simulink model "PowertrainCoolingModel"  (R2020b)
settings: Solver=VariableStepAuto  StartTime=0.0  StopTime=Request.Scaled.Time(end)  MaxStep=1e-1  MinStep=1e-9  RelTol=1e-3
values from neighbouring files (symbols this model uses):
  Accumulator = StraightFinCalculations( Accumulator )    [PowertrainCoolingWrapper.m]
  Controller = StraightFinCalculations( Controller )    [PowertrainCoolingWrapper.m]
  Environment = EnvironmentCalculations( Environment )    [PowertrainCoolingWrapper.m]
  Motor = MotorCalculations( Motor )    [PowertrainCoolingWrapper.m]
  Request = RequestCalculations( Request, Data )    [PowertrainCoolingWrapper.m]
undefined symbols (not defined in the file or in its folder): Chassis, Material
libraries: fl_lib x54, nesl_utility x21
settings Model: Creator=bechr  LastModifiedBy=maxbo
settings SolverCC: InitialStep=1e-9  MaxConsecutiveMinStep=10
settings ModelReferenceCC: ModelReferenceMinAlgLoopOccurrences=on

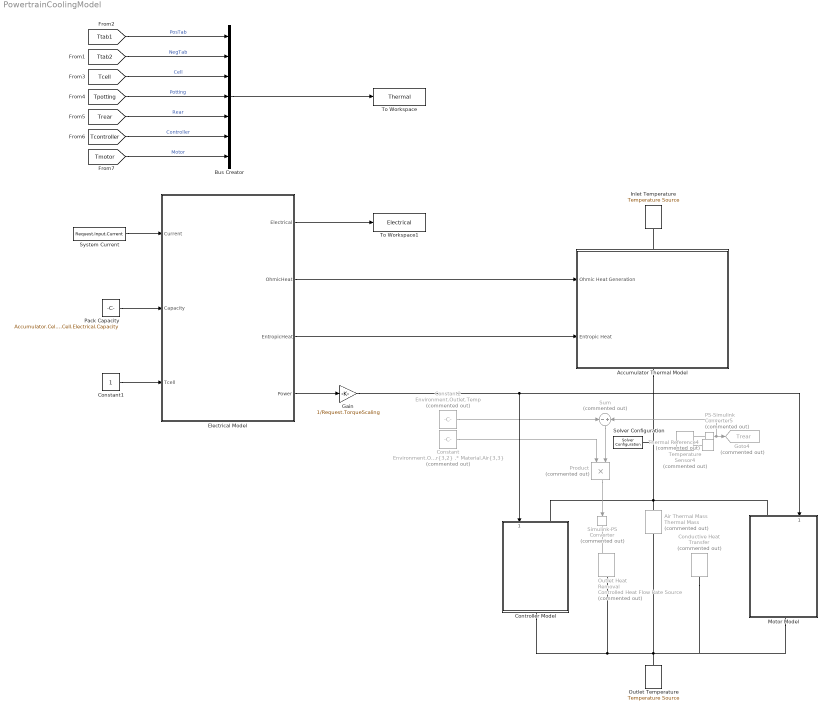
== system PowertrainCoolingModel ==
  Accumulator Thermal Model : Subsystem
      settings: PortSchema="{\"entries\":[{\"content\":{\"sides\":[{\"content\":{\"connectorIds\":[\"LConn1\"]},\"type\":\"ConnectorPlacement.EquallySpacedRectSide\",\"uuid\":\"047de4e7-8380-4083-a16a-e3dcc0474bf0\"},{\"content\":{\"connectorIds\":[\"RConn1\"],\"side\":\"RIGHT\"},\"type\":\"ConnectorPlacement.EquallySpacedRectSide\",\"uuid\":\"fb2ea971-3892-49c2-b754-190bbc105b65\"},{\"content\":{\"connectorIds\":[\"In1\",\"In2\"],\"side\":\"TOP\"},\"type\":\"ConnectorPlacement.EquallySpacedRectSide\",\"uuid\":\"52ae1223-76c9-471f-ad3e-c3ae8e976854\"}]},\"type\":\"ConnectorPlacement.EquallySpacedConnector\",\"uuid\":\"9beae297-ed97-4137-a2f6-556fb11424ca\"}],\"packageUris\":[\"http://schema.mathworks.com/mf0/Connector/19700101\"],\"version\":\"1.0\"}"
  Air Thermal Mass : fl_lib/Thermal/Thermal Elements/Thermal Mass  Commented=on  mass=0.995 .* Chassis.Dimensions.Volume kg  sp_heat=1.0090 kJ/kg/K  T_specify=on  T_priority=High  T=Environment.Outlet.Temp degC  T_nominal_specify=off  T_nominal_unit=K  T_nominal_value=1  Q_specify=off  Q_priority=None  Q=0 W  Q_nominal_specify=off  Q_nominal_unit=W  Q_nominal_value=1
  Bus Creator : BusCreator  Inputs=7
  Conductive Heat Transfer : fl_lib/Thermal/Thermal Elements/Conductive Heat Transfer  Commented=on  area=Chassis.Dimensions.Area m^2  thickness=Chassis.Dimensions.Thickness m  th_cond=Chassis.Thermal.k W/(m*K)  T_specify=off  T_priority=None  T=0 K  T_nominal_specify=off  T_nominal_unit=K  T_nominal_value=1  Q_specify=off  Q_priority=None  Q=0 W  Q_nominal_specify=off  Q_nominal_unit=W  Q_nominal_value=1
  Constant : Constant  Commented=on  Value=Environment.Outlet.FlowRate .* Material.Air{3,2} .* Material.Air{3,3}
  Constant1 : Constant
  Constant2 : Constant  Commented=on  Value=Environment.Outlet.Temp
  Controller Model : Subsystem
      settings: PortSchema="{\"entries\":[{\"content\":{\"sides\":[{\"content\":{\"connectorIds\":[\"LConn1\"]},\"type\":\"ConnectorPlacement.EquallySpacedRectSide\",\"uuid\":\"ee03d1dc-ccff-454a-ba9d-20e22337bc28\"},{\"content\":{\"connectorIds\":[\"In1\",\"RConn1\"],\"side\":\"RIGHT\"},\"type\":\"ConnectorPlacement.EquallySpacedRectSide\",\"uuid\":\"b1e6da54-ab19-4ef3-af09-0565bd1c2c81\"},{\"content\":{\"connectorIds\":[],\"side\":\"TOP\"},\"type\":\"ConnectorPlacement.EquallySpacedRectSide\",\"uuid\":\"cc30cdce-b0f9-4be0-bd93-6142d7ef4c72\"}]},\"type\":\"ConnectorPlacement.EquallySpacedConnector\",\"uuid\":\"1c37dcd3-68ba-409f-82c7-20e952dc67e1\"}],\"packageUris\":[\"http://schema.mathworks.com/mf0/Connector/19700101\"],\"version\":\"1.0\"}"
  Electrical Model : Subsystem
  Gain : Gain  Gain=1/Request.TorqueScaling
  Goto4 : Goto  Commented=on  GotoTag=Trear  TagVisibility=global
  Inlet Temperature : fl_lib/Thermal/Thermal Sources/Temperature Source  temperature=Environment.Inlet.Temp degC
  Motor Model : Subsystem
      settings: PortSchema="{\"entries\":[{\"content\":{\"sides\":[{\"content\":{\"connectorIds\":[\"LConn1\"]},\"type\":\"ConnectorPlacement.EquallySpacedRectSide\",\"uuid\":\"ee03d1dc-ccff-454a-ba9d-20e22337bc28\"},{\"content\":{\"connectorIds\":[\"RConn1\",\"In1\"],\"side\":\"RIGHT\"},\"type\":\"ConnectorPlacement.EquallySpacedRectSide\",\"uuid\":\"b1e6da54-ab19-4ef3-af09-0565bd1c2c81\"},{\"content\":{\"connectorIds\":[],\"side\":\"TOP\"},\"type\":\"ConnectorPlacement.EquallySpacedRectSide\",\"uuid\":\"cc30cdce-b0f9-4be0-bd93-6142d7ef4c72\"}]},\"type\":\"ConnectorPlacement.EquallySpacedConnector\",\"uuid\":\"1c37dcd3-68ba-409f-82c7-20e952dc67e1\"}],\"packageUris\":[\"http://schema.mathworks.com/mf0/Connector/19700101\"],\"version\":\"1.0\"}"
  Outlet Temperature : fl_lib/Thermal/Thermal Sources/Temperature Source  temperature=Environment.Outlet.Temp degC
  Outlet Heat Removal : fl_lib/Thermal/Thermal Sources/Controlled Heat Flow Rate Source  Commented=on
  PS-Simulink Converter5 : nesl_utility/PS-Simulink Converter  Commented=on  PhysicalDomain=network_engine_domain  SubClassName=ps_output  LeftPortType=input  RightPortType=output  PseudoPeriodic=off  Frequencies=[]  Unit=inherit  AffineConversion=off
  Pack Capacity : Constant  Value=Accumulator.Cell.Electrical.NCells .* Accumulator.Cell.Electrical.Capacity
  Product : Product  Commented=on
  Simulink-PS Converter : nesl_utility/Simulink-PS Converter  Commented=on  PhysicalDomain=network_engine_domain  SubClassName=ps_input  LeftPortType=input  RightPortType=output  PseudoPeriodic=off  Frequencies=[]  NoiseDistribution=none  NoiseParameters=[]  Unit=1  AffineConversion=off  FilteringAndDerivatives=provide  SimscapeFilterOrder=1  InputFilterTimeConstant=0.001  UdotUserProvided=0
  Solver Configuration : nesl_utility/Solver Configuration  PhysicalDomain=network_engine_domain  SubClassName=solver  LeftPortType=input  RightPortType=generic  Tones=[]  Harmonics=[]  SimulateNoise=off  Profile=off  UseLocalSampling=off  EnableSwitchedLinearOptims=on  FrequencyDomain=off  UseCCode=off  RelTol=0.001  AbsTol=1e-06  MinStep=1e-09  ToWorkspace=off  RevertToSquareIcSolve=off  NumHomotopyIterations=100  PhasorMode=off  PhasorModeNumHarmonics=1  DoDC=on  ResidualTolerance=1e-09  UseLocalSolver=off  LocalSolverChoice=NE_BACKWARD_EULER_ADVANCER  LocalSolverSampleTime=0.001  DoFixedCost=off  MaxNonlinIter=3  MaxModeIter=2  ComputeImpulses=off  ImpulseIterations=2  LinearAlgebra=auto  EquationFormulation=NE_TIME_EF  DelaysMemoryBudget=1024  AutomaticFiltering=on  FilteringTimeConstant=0.001  PartitionStorageMethod=AS_NEEDED  PartitionMemoryBudget=1024  PartitionMethod=ROBUST
  Sum : Sum  Commented=on  Inputs=-|+
  System Current : FromWorkspace  VariableName=Request.Input.Current  OutputAfterFinalValue=Setting to zero
  Temperature Sensor4 : fl_lib/Thermal/Thermal Sensors/Temperature Sensor  Commented=on
  Thermal Reference4 : fl_lib/Thermal/Thermal Elements/Thermal Reference  Commented=on
  To Workspace : ToWorkspace  VariableName=Thermal  SaveFormat=Timeseries  SampleTime=-1
  To Workspace1 : ToWorkspace  VariableName=Electrical  SaveFormat=Timeseries  SampleTime=-1
  wires:
  [Ttab1] -> Bus Creator/1  "PosTab"
  [Tcell] -> Bus Creator/3  "Cell"
  [Ttab2] -> Bus Creator/2  "NegTab"
  [Tpotting] -> Bus Creator/4  "Potting"
  [Trear] -> Bus Creator/5  "Rear"
  [Tcontroller] -> Bus Creator/6  "Controller"
  [Tmotor] -> Bus Creator/7  "Motor"
  Bus Creator/1 -> To Workspace/1
  Electrical Model/4(Power) -> Gain/1
  System Current/1 -> Electrical Model/1(Current)
  Pack Capacity/1 -> Electrical Model/2(Capacity)
  Electrical Model/1(Electrical) -> To Workspace1/1
  Electrical Model/2(OhmicHeat) -> Accumulator Thermal Model/1(Ohmic Heat Generation)
  Electrical Model/3(EntropicHeat) -> Accumulator Thermal Model/2(" Entropic Heat")
  Constant1/1 -> Electrical Model/3(Tcell)
  Constant2/1 -> Sum/1
  PS-Simulink Converter5/1 -> Sum/2, Goto4/1
  Product/1 -> Simulink-PS Converter/1
  Sum/1 -> Product/2
  Constant/1 -> Product/1
  Gain/1 -> Motor Model/1("Accumulator Power "), Controller Model/1("Accumulator Power ")
  connections:
  Simulink-PS Converter/RConn1 -- Outlet Heat Removal/RConn1
  Outlet Temperature/LConn1 -- Solver Configuration/RConn1 -- Accumulator Thermal Model/RConn1 -- Motor Model/RConn1 -- Controller Model/RConn1 -- Controller Model/LConn1 -- Outlet Heat Removal/LConn1 -- Conductive Heat Transfer/RConn1 -- Motor Model/LConn1
  Thermal Reference4/LConn1 -- Temperature Sensor4/RConn1
  PS-Simulink Converter5/LConn1 -- Temperature Sensor4/RConn2
  Accumulator Thermal Model/LConn1 -- Inlet Temperature/LConn1

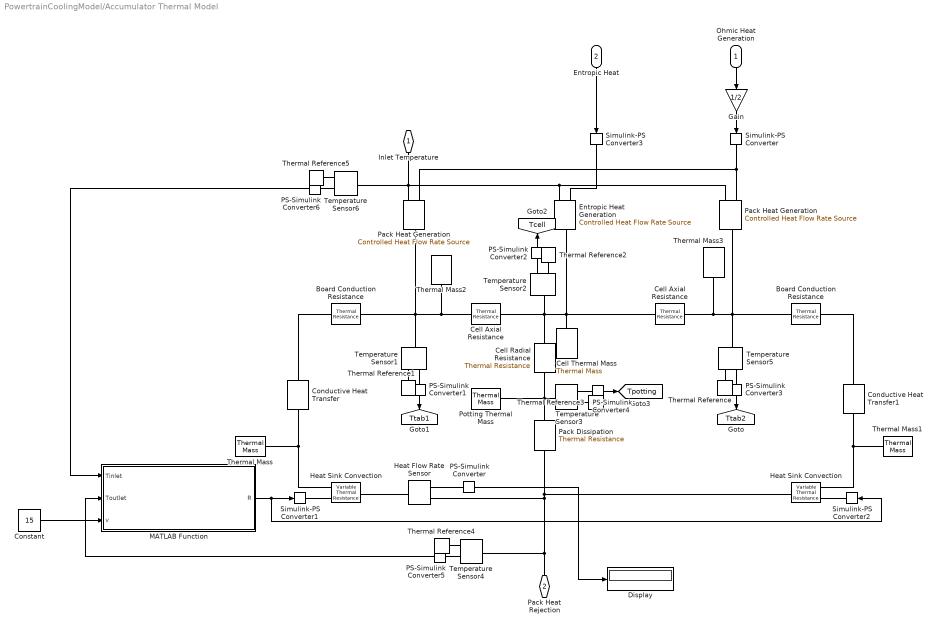
== system PowertrainCoolingModel/Accumulator Thermal Model ==
  Ohmic Heat Generation : Inport
  " Entropic Heat" : Inport  Port=2
  "    Pack Heat Generation" : fl_lib/Thermal/Thermal Sources/Controlled Heat Flow Rate Source
  "  Pack Heat Generation" : fl_lib/Thermal/Thermal Sources/Controlled Heat Flow Rate Source
  Board Conduction Resistance : fl_lib/Thermal/Thermal Elements/Thermal Resistance  resistance=Accumulator.Collector.Thermal.Resistance K/W  T_specify=off  T_priority=None  T=0 K  T_nominal_specify=off  T_nominal_unit=K  T_nominal_value=1  Q_specify=off  Q_priority=None  Q=0 W  Q_nominal_specify=off  Q_nominal_unit=W  Q_nominal_value=1
      settings: SourceProductBaseCode=SS
  "Board Conduction Resistance " : fl_lib/Thermal/Thermal Elements/Thermal Resistance  resistance=1000000 K/W  T_specify=off  T_priority=None  T=0 K  T_nominal_specify=off  T_nominal_unit=K  T_nominal_value=1  Q_specify=off  Q_priority=None  Q=0 W  Q_nominal_specify=off  Q_nominal_unit=W  Q_nominal_value=1
      settings: SourceProductBaseCode=SS
  Cell Axial Resistance : fl_lib/Thermal/Thermal Elements/Thermal Resistance  resistance=Accumulator.Cell.Thermal.R_Axial K/W  T_specify=off  T_priority=None  T=0 K  T_nominal_specify=off  T_nominal_unit=K  T_nominal_value=1  Q_specify=off  Q_priority=None  Q=0 W  Q_nominal_specify=off  Q_nominal_unit=W  Q_nominal_value=1
      settings: SourceProductBaseCode=SS
  "Cell Axial Resistance " : fl_lib/Thermal/Thermal Elements/Thermal Resistance  resistance=Accumulator.Cell.Thermal.R_Axial K/W  T_specify=off  T_priority=None  T=0 K  T_nominal_specify=off  T_nominal_unit=K  T_nominal_value=1  Q_specify=off  Q_priority=None  Q=0 W  Q_nominal_specify=off  Q_nominal_unit=W  Q_nominal_value=1
      settings: SourceProductBaseCode=SS
  Cell Radial Resistance : fl_lib/Thermal/Thermal Elements/Thermal Resistance  resistance=Accumulator.Cell.Thermal.R_Radial K/W  T_specify=off  T_priority=None  T=0 K  T_nominal_specify=off  T_nominal_unit=K  T_nominal_value=1  Q_specify=off  Q_priority=None  Q=0 W  Q_nominal_specify=off  Q_nominal_unit=W  Q_nominal_value=1
      settings: SourceProductBaseCode=SS
  Cell Thermal Mass : fl_lib/Thermal/Thermal Elements/Thermal Mass  mass=Accumulator.Cell.Electrical.NCells .* Accumulator.Cell.Mass.m kg  sp_heat=Accumulator.Cell.Thermal.cp kJ/kg/K  T_specify=on  T_priority=Low  T=Environment.Inlet.Temp degC  T_nominal_specify=off  T_nominal_unit=K  T_nominal_value=1  Q_specify=off  Q_priority=None  Q=0 W  Q_nominal_specify=off  Q_nominal_unit=W  Q_nominal_value=1
  Conductive Heat Transfer : fl_lib/Thermal/Thermal Elements/Conductive Heat Transfer  area=Accumulator.Fin.Dimensions.Width * Accumulator.Fin.Dimensions.Length * 5 m^2  thickness=0.2 mm  th_cond=1.6 W/(m*K)  T_specify=off  T_priority=None  T=0 K  T_nominal_specify=off  T_nominal_unit=K  T_nominal_value=1  Q_specify=off  Q_priority=None  Q=0 W  Q_nominal_specify=off  Q_nominal_unit=W  Q_nominal_value=1
  Conductive Heat Transfer1 : fl_lib/Thermal/Thermal Elements/Conductive Heat Transfer  area=Accumulator.Fin.Dimensions.Width * Accumulator.Fin.Dimensions.Length * 5 m^2  thickness=0.2 mm  th_cond=1.6 W/(m*K)  T_specify=off  T_priority=None  T=0 K  T_nominal_specify=off  T_nominal_unit=K  T_nominal_value=1  Q_specify=off  Q_priority=None  Q=0 W  Q_nominal_specify=off  Q_nominal_unit=W  Q_nominal_value=1
  Constant : Constant  Value=15
  Display : Display
  Entropic Heat Generation : fl_lib/Thermal/Thermal Sources/Controlled Heat Flow Rate Source
  Gain : Gain  Gain=1/2
  Heat Flow Rate Sensor : fl_lib/Thermal/Thermal Sensors/Heat Flow Rate Sensor
      settings: SourceProductBaseCode=SS
  Heat Sink Convection : fl_lib/Thermal/Thermal Elements/Variable Thermal Resistance  R_min=0 K/W  T_specify=off  T_priority=None  T=0 K  T_nominal_specify=off  T_nominal_unit=K  T_nominal_value=1  Q_specify=off  Q_priority=None  Q=0 W  Q_nominal_specify=off  Q_nominal_unit=W  Q_nominal_value=1
      settings: SourceProductBaseCode=SS  InternalSimscapePortConfiguration="{\"Bottom\":[],\"Left\":[{\"id\":\"A\",\"label\":\"A\",\"type\":\"foundation.thermal.thermal\"},{\"id\":\"R\",\"label\":\"R\",\"type\":\"input\"}],\"Right\":[{\"id\":\"B\",\"label\":\"B\",\"type\":\"foundation.thermal.thermal\"}],\"Top\":[]}"
  "Heat Sink Convection " : fl_lib/Thermal/Thermal Elements/Variable Thermal Resistance  R_min=0 K/W  T_specify=off  T_priority=None  T=0 K  T_nominal_specify=off  T_nominal_unit=K  T_nominal_value=1  Q_specify=off  Q_priority=None  Q=0 W  Q_nominal_specify=off  Q_nominal_unit=W  Q_nominal_value=1
      settings: SourceProductBaseCode=SS  InternalSimscapePortConfiguration="{\"Bottom\":[],\"Left\":[{\"id\":\"A\",\"label\":\"A\",\"type\":\"foundation.thermal.thermal\"},{\"id\":\"R\",\"label\":\"R\",\"type\":\"input\"}],\"Right\":[{\"id\":\"B\",\"label\":\"B\",\"type\":\"foundation.thermal.thermal\"}],\"Top\":[]}"
  MATLAB Function : MATLAB Function  TreatAsAtomicUnit=on
  PS-Simulink Converter{,1..6} (7 alike) : nesl_utility/PS-Simulink Converter  PhysicalDomain=network_engine_domain  SubClassName=ps_output  LeftPortType=input  RightPortType=output  PseudoPeriodic=off  Frequencies=[]  Unit=inherit  AffineConversion=off
  Pack Dissipation : fl_lib/Thermal/Thermal Elements/Thermal Resistance  resistance=1E6 K/W  T_specify=off  T_priority=None  T=0 K  T_nominal_specify=off  T_nominal_unit=K  T_nominal_value=1  Q_specify=off  Q_priority=None  Q=0 W  Q_nominal_specify=off  Q_nominal_unit=W  Q_nominal_value=1
      settings: SourceProductBaseCode=SS
  Potting Thermal Mass : fl_lib/Thermal/Thermal Elements/Thermal Mass  mass=Accumulator.Potting.Mass.m kg  sp_heat=Accumulator.Potting.Thermal.cp kJ/kg/K  T_specify=on  T_priority=Low  T=Environment.Inlet.Temp degC  T_nominal_specify=off  T_nominal_unit=K  T_nominal_value=1  Q_specify=off  Q_priority=None  Q=0 W  Q_nominal_specify=off  Q_nominal_unit=W  Q_nominal_value=1
  Simulink-PS Converter{,1..3} (4 alike) : nesl_utility/Simulink-PS Converter  PhysicalDomain=network_engine_domain  SubClassName=ps_input  LeftPortType=input  RightPortType=output  PseudoPeriodic=off  Frequencies=[]  NoiseDistribution=none  NoiseParameters=[]  Unit=1  AffineConversion=off  FilteringAndDerivatives=provide  SimscapeFilterOrder=1  InputFilterTimeConstant=0.001  UdotUserProvided=0
  Temperature Sensor{1..6} (6 alike) : fl_lib/Thermal/Thermal Sensors/Temperature Sensor
  Thermal Mass : fl_lib/Thermal/Thermal Elements/Thermal Mass  mass=1.16 / 2 * 5 kg  sp_heat=900 J/kg/K  T_specify=off  T_priority=High  T=300 K  T_nominal_specify=off  T_nominal_unit=K  T_nominal_value=1  Q_specify=off  Q_priority=None  Q=0 W  Q_nominal_specify=off  Q_nominal_unit=W  Q_nominal_value=1
  Thermal Mass1 : fl_lib/Thermal/Thermal Elements/Thermal Mass  mass=1.16 / 2 * 5 kg  sp_heat=900 J/kg/K  T_specify=off  T_priority=High  T=300 K  T_nominal_specify=off  T_nominal_unit=K  T_nominal_value=1  Q_specify=off  Q_priority=None  Q=0 W  Q_nominal_specify=off  Q_nominal_unit=W  Q_nominal_value=1
  Thermal Mass2 : fl_lib/Thermal/Thermal Elements/Thermal Mass  mass=2 * Accumulator.Cell.Electrical.NCells g  sp_heat=475 J/kg/K  T_specify=off  T_priority=High  T=300 K  T_nominal_specify=off  T_nominal_unit=K  T_nominal_value=1  Q_specify=off  Q_priority=None  Q=0 W  Q_nominal_specify=off  Q_nominal_unit=W  Q_nominal_value=1
  Thermal Mass3 : fl_lib/Thermal/Thermal Elements/Thermal Mass  mass=2 * Accumulator.Cell.Electrical.NCells g  sp_heat=475 J/kg/K  T_specify=off  T_priority=High  T=300 K  T_nominal_specify=off  T_nominal_unit=K  T_nominal_value=1  Q_specify=off  Q_priority=None  Q=0 W  Q_nominal_specify=off  Q_nominal_unit=W  Q_nominal_value=1
  Thermal Reference{,1..5} (6 alike) : fl_lib/Thermal/Thermal Elements/Thermal Reference
  " Inlet Temperature" : PMIOPort  Side=Left
  Pack Heat Rejection : PMIOPort  Port=2  Side=Right
  tag scope: Tcell=global, Tpotting=global, Ttab1=global, Ttab2=global
  wires:
  PS-Simulink Converter4/1 -> [Tpotting]
  PS-Simulink Converter3/1 -> [Ttab2]
  PS-Simulink Converter2/1 -> [Tcell]
  PS-Simulink Converter1/1 -> [Ttab1]
  Ohmic Heat Generation/1 -> Gain/1
  Gain/1 -> Simulink-PS Converter/1
  MATLAB Function/1(R) -> Simulink-PS Converter2/1, Simulink-PS Converter1/1
  PS-Simulink Converter5/1 -> MATLAB Function/2(Toutlet)
  PS-Simulink Converter6/1 -> MATLAB Function/1(Tinlet)
  Constant/1 -> MATLAB Function/3(v)
  " Entropic Heat"/1 -> Simulink-PS Converter3/1
  PS-Simulink Converter/1 -> Display/1
  connections:
  Temperature Sensor2/LConn1 -- Entropic Heat Generation/LConn1 -- Cell Thermal Mass/LConn1 -- "Cell Axial Resistance "/RConn1 -- Cell Radial Resistance/LConn1 -- Cell Axial Resistance/RConn1
  Temperature Sensor3/LConn1 -- Cell Radial Resistance/RConn1 -- Pack Dissipation/LConn1 -- Potting Thermal Mass/LConn1
  Conductive Heat Transfer/LConn1 -- Board Conduction Resistance/RConn1
  Heat Sink Convection/LConn1 -- Conductive Heat Transfer/RConn1 -- Thermal Mass/LConn1
  Thermal Reference1/LConn1 -- Temperature Sensor1/RConn1
  Temperature Sensor1/LConn1 -- Cell Axial Resistance/LConn1 -- Thermal Mass2/LConn1 -- "    Pack Heat Generation"/LConn1 -- Board Conduction Resistance/LConn1
  "Heat Sink Convection "/LConn1 -- Conductive Heat Transfer1/RConn1 -- Thermal Mass1/LConn1
  "    Pack Heat Generation"/RConn2 -- " Inlet Temperature"/RConn1 -- "  Pack Heat Generation"/RConn2 -- Entropic Heat Generation/RConn2 -- Temperature Sensor6/LConn1
  PS-Simulink Converter2/LConn1 -- Temperature Sensor2/RConn2
  "  Pack Heat Generation"/LConn1 -- Thermal Mass3/LConn1 -- "Cell Axial Resistance "/LConn1 -- Temperature Sensor5/LConn1 -- "Board Conduction Resistance "/LConn1
  PS-Simulink Converter3/LConn1 -- Temperature Sensor5/RConn2
  Thermal Reference/LConn1 -- Temperature Sensor5/RConn1
  Pack Dissipation/RConn1 -- Heat Flow Rate Sensor/RConn2 -- Temperature Sensor4/LConn1 -- Pack Heat Rejection/RConn1 -- "Heat Sink Convection "/RConn1
  "    Pack Heat Generation"/RConn1 -- Simulink-PS Converter/RConn1 -- "  Pack Heat Generation"/RConn1
  Conductive Heat Transfer1/LConn1 -- "Board Conduction Resistance "/RConn1
  PS-Simulink Converter4/LConn1 -- Temperature Sensor3/RConn2
  Thermal Reference3/LConn1 -- Temperature Sensor3/RConn1
  PS-Simulink Converter1/LConn1 -- Temperature Sensor1/RConn2
  Thermal Reference2/LConn1 -- Temperature Sensor2/RConn1
  Simulink-PS Converter1/RConn1 -- Heat Sink Convection/LConn2
  Thermal Reference4/LConn1 -- Temperature Sensor4/RConn1
  PS-Simulink Converter5/LConn1 -- Temperature Sensor4/RConn2
  PS-Simulink Converter6/LConn1 -- Temperature Sensor6/RConn2
  Thermal Reference5/LConn1 -- Temperature Sensor6/RConn1
  Simulink-PS Converter2/RConn1 -- "Heat Sink Convection "/LConn2
  Simulink-PS Converter3/RConn1 -- Entropic Heat Generation/RConn1
  Heat Flow Rate Sensor/LConn1 -- Heat Sink Convection/RConn1
  PS-Simulink Converter/LConn1 -- Heat Flow Rate Sensor/RConn1

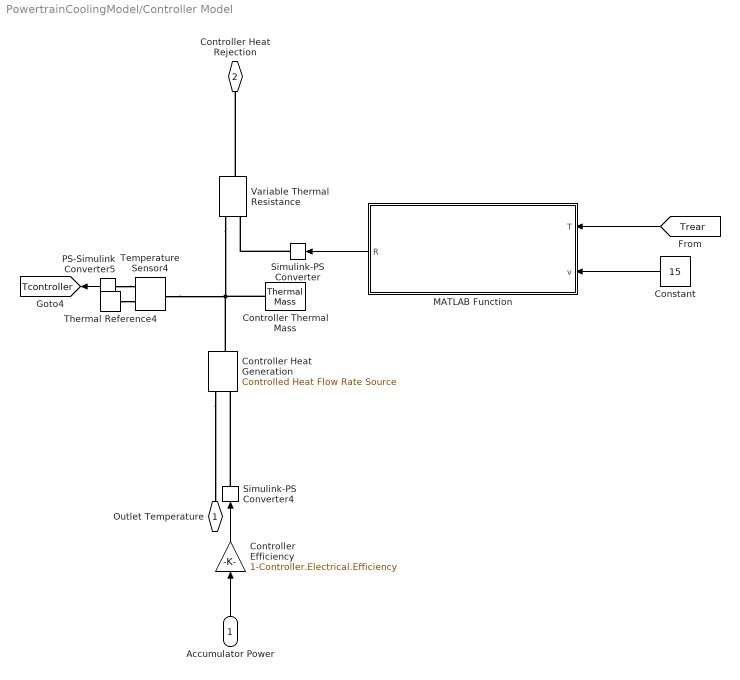
== system PowertrainCoolingModel/Controller Model ==
  "Accumulator Power " : Inport
  Constant : Constant  Value=15
  Controller Efficiency : Gain  Gain=1-Controller.Electrical.Efficiency
  Controller Heat Generation : fl_lib/Thermal/Thermal Sources/Controlled Heat Flow Rate Source
  Controller Thermal Mass : fl_lib/Thermal/Thermal Elements/Thermal Mass  mass=1 kg  sp_heat=2.2137e+03 J/kg/K  T_specify=on  T_priority=None  T=Environment.Outlet.Temp degC  T_nominal_specify=off  T_nominal_unit=K  T_nominal_value=1  Q_specify=off  Q_priority=None  Q=0 W  Q_nominal_specify=off  Q_nominal_unit=W  Q_nominal_value=1
  MATLAB Function : MATLAB Function  TreatAsAtomicUnit=on
  PS-Simulink Converter5 : nesl_utility/PS-Simulink Converter  PhysicalDomain=network_engine_domain  SubClassName=ps_output  LeftPortType=input  RightPortType=output  PseudoPeriodic=off  Frequencies=[]  Unit=inherit  AffineConversion=off
  Simulink-PS Converter : nesl_utility/Simulink-PS Converter  PhysicalDomain=network_engine_domain  SubClassName=ps_input  LeftPortType=input  RightPortType=output  PseudoPeriodic=off  Frequencies=[]  NoiseDistribution=none  NoiseParameters=[]  Unit=1  AffineConversion=off  FilteringAndDerivatives=provide  SimscapeFilterOrder=1  InputFilterTimeConstant=0.001  UdotUserProvided=0
  Simulink-PS Converter4 : nesl_utility/Simulink-PS Converter  PhysicalDomain=network_engine_domain  SubClassName=ps_input  LeftPortType=input  RightPortType=output  PseudoPeriodic=off  Frequencies=[]  NoiseDistribution=none  NoiseParameters=[]  Unit=1  AffineConversion=off  FilteringAndDerivatives=provide  SimscapeFilterOrder=1  InputFilterTimeConstant=0.001  UdotUserProvided=0
  Temperature Sensor4 : fl_lib/Thermal/Thermal Sensors/Temperature Sensor
  Thermal Reference4 : fl_lib/Thermal/Thermal Elements/Thermal Reference
  Variable Thermal Resistance : fl_lib/Thermal/Thermal Elements/Variable Thermal Resistance  R_min=0 K/W  T_specify=off  T_priority=None  T=0 K  T_nominal_specify=off  T_nominal_unit=K  T_nominal_value=1  Q_specify=off  Q_priority=None  Q=0 W  Q_nominal_specify=off  Q_nominal_unit=W  Q_nominal_value=1
      settings: SourceProductBaseCode=SS  InternalSimscapePortConfiguration="{\"Bottom\":[],\"Left\":[{\"id\":\"A\",\"label\":\"A\",\"type\":\"foundation.thermal.thermal\"},{\"id\":\"R\",\"label\":\"R\",\"type\":\"input\"}],\"Right\":[{\"id\":\"B\",\"label\":\"B\",\"type\":\"foundation.thermal.thermal\"}],\"Top\":[]}"
  Outlet Temperature : PMIOPort  Side=Left
  Controller Heat Rejection : PMIOPort  Port=2  Side=Right
  tag scope: Tcontroller=global
  wires:
  PS-Simulink Converter5/1 -> [Tcontroller]
  "Accumulator Power "/1 -> Controller Efficiency/1
  Controller Efficiency/1 -> Simulink-PS Converter4/1
  Constant/1 -> MATLAB Function/2(v)
  [Trear] -> MATLAB Function/1(T)
  MATLAB Function/1(R) -> Simulink-PS Converter/1
  connections:
  Controller Heat Generation/LConn1 -- Variable Thermal Resistance/LConn1 -- Temperature Sensor4/LConn1 -- Controller Thermal Mass/LConn1
  Simulink-PS Converter4/RConn1 -- Controller Heat Generation/RConn1
  Variable Thermal Resistance/RConn1 -- Controller Heat Rejection/RConn1
  Controller Heat Generation/RConn2 -- Outlet Temperature/RConn1
  PS-Simulink Converter5/LConn1 -- Temperature Sensor4/RConn2
  Thermal Reference4/LConn1 -- Temperature Sensor4/RConn1
  Simulink-PS Converter/RConn1 -- Variable Thermal Resistance/LConn2

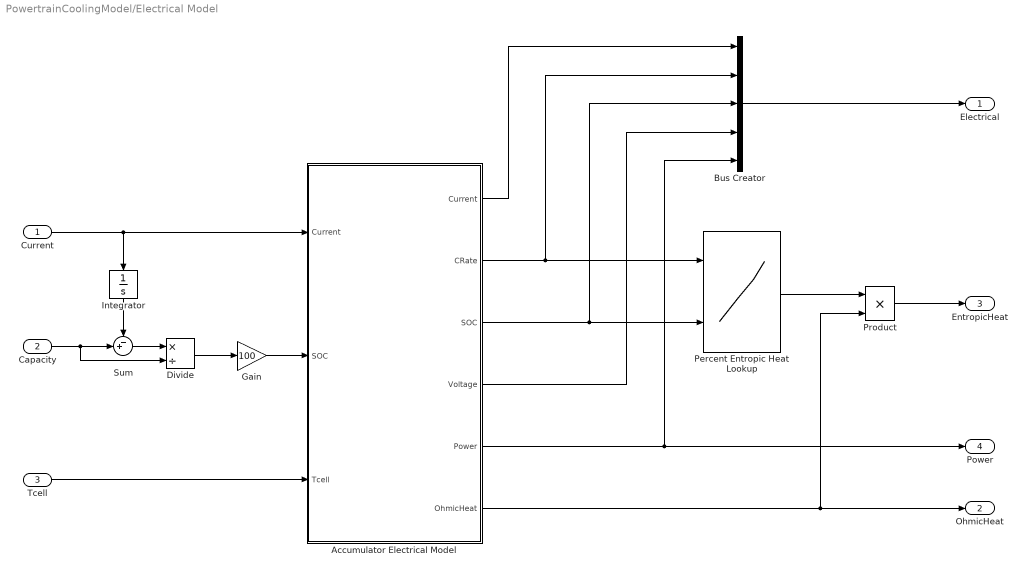
== system PowertrainCoolingModel/Electrical Model ==
  Current : Inport
  Capacity : Inport  Port=2
  Tcell : Inport  Port=3
  Accumulator Electrical Model : MATLAB Function  TreatAsAtomicUnit=on
  Bus Creator : BusCreator  Inputs=5
  Divide : Product  Inputs=*/
  Gain : Gain  Gain=100
  Integrator : Integrator
  Percent Entropic Heat Lookup : Lookup_n-D  BreakpointsForDimension1=Accumulator.Cell.Thermal.EntropyData.CRate  BreakpointsForDimension2=Accumulator.Cell.Thermal.EntropyData.SOC  BeginIndexSearchUsingPreviousIndexResult=on  Table=Accumulator.Cell.Thermal.EntropyData.PerEntropy  ExtrapMethod=Clip  DiagnosticForOutOfRangeInput=Warning  InternalRulePriority=Speed  RndMeth=Simplest  InputSameDT=on
      settings: InputPortMap=u0,u1
  Product : Product
  Sum : Sum  Inputs=-+|
  Electrical : Outport
  OhmicHeat : Outport  Port=2
  EntropicHeat : Outport  Port=3
  Power : Outport  Port=4
  wires:
  Accumulator Electrical Model/1(Current) -> Bus Creator/1
  Integrator/1 -> Sum/1
  Tcell/1 -> Accumulator Electrical Model/3(Tcell)
  Accumulator Electrical Model/6(OhmicHeat) -> Product/2, OhmicHeat/1
  Accumulator Electrical Model/2(CRate) -> Bus Creator/2, Percent Entropic Heat Lookup/1
  Capacity/1 -> Divide/2, Sum/2
  Accumulator Electrical Model/5(Power) -> Bus Creator/5, Power/1
  Current/1 -> Integrator/1, Accumulator Electrical Model/1("Current ")
  Accumulator Electrical Model/3(SOC) -> Bus Creator/3, Percent Entropic Heat Lookup/2
  Product/1 -> EntropicHeat/1
  Percent Entropic Heat Lookup/1 -> Product/1
  Accumulator Electrical Model/4(Voltage) -> Bus Creator/4
  Bus Creator/1 -> Electrical/1
  Sum/1 -> Divide/1
  Divide/1 -> Gain/1
  Gain/1 -> Accumulator Electrical Model/2("SOC ")

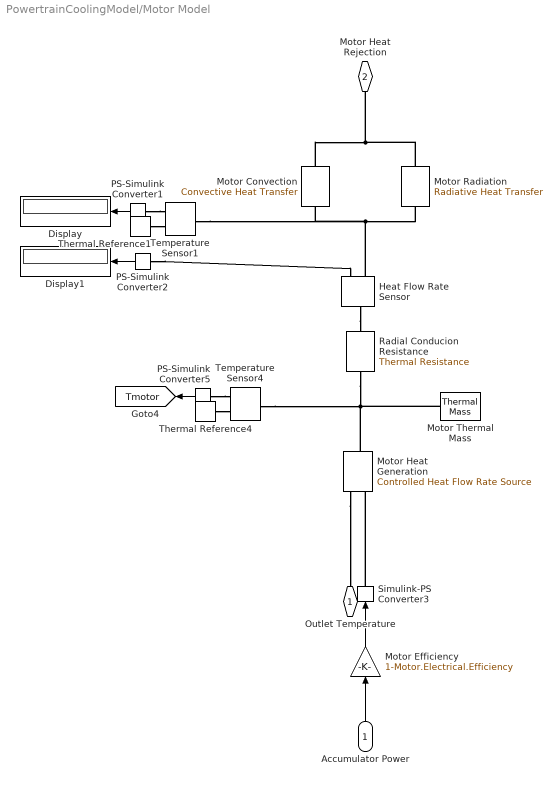
== system PowertrainCoolingModel/Motor Model ==
  "Accumulator Power " : Inport
  " Motor Heat Generation" : fl_lib/Thermal/Thermal Sources/Controlled Heat Flow Rate Source
  Display : Display
  Display1 : Display
  Heat Flow Rate Sensor : fl_lib/Thermal/Thermal Sensors/Heat Flow Rate Sensor
      settings: SourceProductBaseCode=SS
  Motor Convection : fl_lib/Thermal/Thermal Elements/Convective Heat Transfer  area=Motor.Dimensions.A m^2  heat_tr_coeff=Motor.Thermal.h W/(m^2 * K)  T_specify=off  T_priority=None  T=0 K  T_nominal_specify=off  T_nominal_unit=K  T_nominal_value=1  Q_specify=off  Q_priority=None  Q=0 W  Q_nominal_specify=off  Q_nominal_unit=W  Q_nominal_value=1
  Motor Efficiency : Gain  Gain=1-Motor.Electrical.Efficiency
  Motor Radiation : fl_lib/Thermal/Thermal Elements/Radiative Heat Transfer  area=Motor.Dimensions.A m^2  rad_tr_coeff=Motor.Thermal.eps W/(m^2*K^4)  T_specify=off  T_priority=None  T=0 K  T_nominal_specify=off  T_nominal_unit=K  T_nominal_value=1  Q_specify=off  Q_priority=None  Q=0 W  Q_nominal_specify=off  Q_nominal_unit=W  Q_nominal_value=1
      settings: SourceProductBaseCode=SS  InternalSimscapePortConfiguration="{\"Bottom\":[],\"Left\":[{\"id\":\"A\",\"label\":\"A\",\"type\":\"foundation.thermal.thermal\"}],\"Right\":[{\"id\":\"B\",\"label\":\"B\",\"type\":\"foundation.thermal.thermal\"}],\"Top\":[]}"
  Motor Thermal Mass : fl_lib/Thermal/Thermal Elements/Thermal Mass  mass=Motor.Mass.m kg  sp_heat=Motor.Thermal.cp kJ/kg/K  T_specify=on  T_priority=High  T=Environment.Outlet.Temp degC  T_nominal_specify=off  T_nominal_unit=K  T_nominal_value=1  Q_specify=off  Q_priority=None  Q=0 W  Q_nominal_specify=off  Q_nominal_unit=W  Q_nominal_value=1
  PS-Simulink Converter1 : nesl_utility/PS-Simulink Converter  PhysicalDomain=network_engine_domain  SubClassName=ps_output  LeftPortType=input  RightPortType=output  PseudoPeriodic=off  Frequencies=[]  Unit=inherit  AffineConversion=off
  PS-Simulink Converter2 : nesl_utility/PS-Simulink Converter  PhysicalDomain=network_engine_domain  SubClassName=ps_output  LeftPortType=input  RightPortType=output  PseudoPeriodic=off  Frequencies=[]  Unit=inherit  AffineConversion=off
  PS-Simulink Converter5 : nesl_utility/PS-Simulink Converter  PhysicalDomain=network_engine_domain  SubClassName=ps_output  LeftPortType=input  RightPortType=output  PseudoPeriodic=off  Frequencies=[]  Unit=inherit  AffineConversion=off
  Radial Conducion Resistance : fl_lib/Thermal/Thermal Elements/Thermal Resistance  resistance=0.01 K/W  T_specify=off  T_priority=None  T=0 K  T_nominal_specify=off  T_nominal_unit=K  T_nominal_value=1  Q_specify=off  Q_priority=None  Q=0 W  Q_nominal_specify=off  Q_nominal_unit=W  Q_nominal_value=1
      settings: SourceProductBaseCode=SS
  Simulink-PS Converter3 : nesl_utility/Simulink-PS Converter  PhysicalDomain=network_engine_domain  SubClassName=ps_input  LeftPortType=input  RightPortType=output  PseudoPeriodic=off  Frequencies=[]  NoiseDistribution=none  NoiseParameters=[]  Unit=1  AffineConversion=off  FilteringAndDerivatives=provide  SimscapeFilterOrder=1  InputFilterTimeConstant=0.001  UdotUserProvided=0
  Temperature Sensor1 : fl_lib/Thermal/Thermal Sensors/Temperature Sensor
  Temperature Sensor4 : fl_lib/Thermal/Thermal Sensors/Temperature Sensor
  Thermal Reference1 : fl_lib/Thermal/Thermal Elements/Thermal Reference
  Thermal Reference4 : fl_lib/Thermal/Thermal Elements/Thermal Reference
  Outlet Temperature : PMIOPort  Side=Left
  "Motor Heat Rejection " : PMIOPort  Port=2  Side=Right
  tag scope: Tmotor=global
  wires:
  "Accumulator Power "/1 -> Motor Efficiency/1
  PS-Simulink Converter5/1 -> [Tmotor]
  Motor Efficiency/1 -> Simulink-PS Converter3/1
  PS-Simulink Converter1/1 -> Display/1
  PS-Simulink Converter2/1 -> Display1/1
  connections:
  " Motor Heat Generation"/RConn2 -- Outlet Temperature/RConn1
  " Motor Heat Generation"/LConn1 -- Radial Conducion Resistance/LConn1 -- Temperature Sensor4/LConn1 -- Motor Thermal Mass/LConn1
  Simulink-PS Converter3/RConn1 -- " Motor Heat Generation"/RConn1
  Motor Radiation/RConn1 -- Motor Convection/RConn1 -- "Motor Heat Rejection "/RConn1
  PS-Simulink Converter5/LConn1 -- Temperature Sensor4/RConn2
  Thermal Reference4/LConn1 -- Temperature Sensor4/RConn1
  Temperature Sensor1/LConn1 -- Motor Convection/LConn1 -- Heat Flow Rate Sensor/RConn2 -- Motor Radiation/LConn1
  PS-Simulink Converter1/LConn1 -- Temperature Sensor1/RConn2
  Thermal Reference1/LConn1 -- Temperature Sensor1/RConn1
  Heat Flow Rate Sensor/LConn1 -- Radial Conducion Resistance/RConn1
  PS-Simulink Converter2/LConn1 -- Heat Flow Rate Sensor/RConn1

== matlab function PowertrainCoolingModel/Accumulator Thermal Model/MATLAB Function ==
  data: Tinlet input; R output; Toutlet input; v input; Parameter parameter
function R = PackConvectionResistanceEstimation(Tinlet, Toutlet, v, Parameter)

%%% Find Average Temperature
T = (Tinlet + Toutlet) / 2;

%%% Evaluate Air Properties
if Parameter.Material.Air(1,1) < T && T < Parameter.Material.Air(end,1) 
    rho = interp1( Parameter.Material.Air(:,1), Parameter.Material.Air(:,2), T );
    cp  = interp1( Parameter.Material.Air(:,1), Parameter.Material.Air(:,3), T );
    mu  = interp1( Parameter.Material.Air(:,1), Parameter.Material.Air(:,4), T );
    k   = interp1( Parameter.Material.Air(:,1), Parameter.Material.Air(:,5), T );
    Pr  = interp1( Parameter.Material.Air(:,1), Parameter.Material.Air(:,6), T );
else
    rho = Parameter.Material.Air(end,2);
    cp  = Parameter.Material.Air(end,3);
    mu  = Parameter.Material.Air(end,4);
    k   = Parameter.Material.Air(end,5);
    Pr  = Parameter.Material.Air(end,6);
end

%%% Heat Transfer Correlations
    % Source: https://www.electronics-cooling.com/2003/02/estimating-parallel-plate-fin-heat-sink-thermal-resistance/
    
Re = rho .* v .* Parameter.Accumulator.Fin.Dimensions.Spacing^2 ./ ...
    ( mu .* Parameter.Accumulator.Fin.Dimensions.Length );

Nu_b = ( 1 ./ ( Re .* Pr / 2 ).^3 + ...
    1 ./ ( 0.664 .* sqrt(Re) .* Pr.^(0.33) .* sqrt( 1 + 3.65./sqrt(Re) ) ).^3 ).^(-0.33); 

h = Nu_b .* k ./ Parameter.Accumulator.Fin.Dimensions.Spacing;

m = sqrt( 2 .* h ./ (Parameter.Accumulator.Fin.Thermal.k .* Parameter.Accumulator.Fin.Dimensions.Thick) );

eta_f = tanh( m * Parameter.Accumulator.Fin.Dimensions.Height ) ./ (m .* Parameter.Accumulator.Fin.Dimensions.Height);

R_hs = 1 ./ ( h .* ( 5* Parameter.Accumulator.Fin.Dimensions.Abase + ...
    Parameter.Accumulator.Cell.Electrical.NSubpacks * Parameter.Accumulator.Fin.Dimensions.N .* eta_f .* Parameter.Accumulator.Fin.Dimensions.Afin ) );

R = R_hs + Parameter.Accumulator.Fin.Dimensions.Base ./ ...
    ( Parameter.Accumulator.Cell.Electrical.NSubpacks * Parameter.Accumulator.Fin.Thermal.k .* Parameter.Accumulator.Fin.Dimensions.Width .* Parameter.Accumulator.Fin.Dimensions.Length );

== matlab function PowertrainCoolingModel/Controller Model/MATLAB Function ==
  data: T input; R output; v input; Parameter parameter
function R = PackConvectionResistanceEstimation(T, v, Parameter)

%%% Evaluate Air Properties
if Parameter.Material.Air(1,1) < T && T < Parameter.Material.Air(end,1) 
    rho = interp1( Parameter.Material.Air(:,1), Parameter.Material.Air(:,2), T );
    cp  = interp1( Parameter.Material.Air(:,1), Parameter.Material.Air(:,3), T );
    mu  = interp1( Parameter.Material.Air(:,1), Parameter.Material.Air(:,4), T );
    k   = interp1( Parameter.Material.Air(:,1), Parameter.Material.Air(:,5), T );
    Pr  = interp1( Parameter.Material.Air(:,1), Parameter.Material.Air(:,6), T );
else
    rho = Parameter.Material.Air(end,2);
    cp  = Parameter.Material.Air(end,3);
    mu  = Parameter.Material.Air(end,4);
    k   = Parameter.Material.Air(end,5);
    Pr  = Parameter.Material.Air(end,6);
end

%%% Heat Transfer Correlations
    % Source: https://www.electronics-cooling.com/2003/02/estimating-parallel-plate-fin-heat-sink-thermal-resistance/ 
    
Re = rho .* v .* Parameter.Controller.Fin.Dimensions.Spacing^2 ./ ...
    ( mu .* Parameter.Controller.Fin.Dimensions.Length );

Nu_b = ( 1 ./ ( Re .* Pr / 2 ).^3 + ...
    1 ./ ( 0.664 .* sqrt(Re) .* Pr.^(0.33) .* sqrt( 1 + 3.65./sqrt(Re) ) ).^3 ).^(-0.33); 

h = 11.8;
%h = Nu_b .* k ./ Parameter.Controller.Fin.Dimensions.Spacing;

m = sqrt( 2 .* h ./ (Parameter.Controller.Fin.Thermal.k .* Parameter.Controller.Fin.Dimensions.Thick) );

eta_f = tanh( m * Parameter.Controller.Fin.Dimensions.Height ) ./ (m .* Parameter.Controller.Fin.Dimensions.Height);

R_hs = 1 ./ ( h .* ( Parameter.Controller.Fin.Dimensions.Abase + ...
    Parameter.Controller.Fin.Dimensions.N .* eta_f .* Parameter.Controller.Fin.Dimensions.Afin ) );

R = R_hs + Parameter.Controller.Fin.Dimensions.Base ./ ...
    ( Parameter.Controller.Fin.Thermal.k .* Parameter.Controller.Fin.Dimensions.Width .* Parameter.Controller.Fin.Dimensions.Length );

== matlab function PowertrainCoolingModel/Electrical Model/Accumulator Electrical Model ==
  data: Current output; CRate output; SOC output; Voltage output; Power output; OhmicHeat output; Current input; SOC input; Tcell input; Parameter parameter
function [Current, CRate, SOC, Voltage, Power, OhmicHeat] = ...
    AccumulatorElectricalModel(Current, SOC, Tcell, Parameter)

    %%% C-Rate Calculation
    Capacity = Parameter.Accumulator.Cell.Electrical.Capacity / (3600);
        % Pack Capacity [A-h]

    CRate = abs(Current) / (Capacity .* Parameter.Accumulator.Cell.Electrical.NParallel);

    %%% Internal Resistance Lookup
    IR = Parameter.Accumulator.Cell.Electrical.Model.IR .* ...
        Parameter.Accumulator.Cell.Electrical.NSeries ./ Parameter.Accumulator.Cell.Electrical.NParallel;

    %%% Ohmic Heat Generation
    OhmicHeat = Current.^2 .* IR;

    %%% Voltage Lookup
    Voltage = Parameter.Accumulator.Cell.Electrical.Model.OCV .* Parameter.Accumulator.Cell.Electrical.NSeries;

    %%% Power Generation
    Power = Parameter.Controller.TorqueScaling .* Current .* Voltage;
